simulink model "HmfCraneMbsModel"  (R2024b)
settings: Solver=FixedStepAuto  StartTime=0.0  StopTime=1  FixedStep=0.001  MaxStep=0.005  RelTol=1e-3
undefined symbols (not defined in the file): thetaList0, X, Y, Z
libraries: sm_lib x75, fl_lib x15, nesl_utility x12
(part 1 of 2)
settings Model: Creator=sindr  LastModifiedBy=hagen
settings RTWCC: GPUComputeCapability=3.5
settings ExplorerConfigSet: InternalSimMechanicsExplorerSettings="<ExplorerConfiguration><canonicalview>default</canonicalview><AnimationSetting><BasePlaybackSpeed>1.0</BasePlaybackSpeed><PlaybackSpeedFactor>1.0</PlaybackSpeedFactor></AnimationSetting><TilePanel><TileInfo><Tiles Columns=\"1\" Count=\"1\" Rows=\"1\"><Column Weight=\"1\"/><Row Weight=\"1\"/><Tile Height=\"1\" Width=\"1\" X=\"0\" Y=\"0\"/></Tiles></TileInfo><SceneInfo><SceneViewer><BGColor><R>0.800000011920928955</R><G>0.800000011920928955</G><B>0.800000011920928955</B></BGColor><Camera><DoPerspective>off</DoPerspective><Position><X>4.53532304319928414</X><Y>-3.6203597502527578</Y><Z>2.5915310173647752</Z></Position><Center><X>-0.318270324932377058</X><Y>2.33029046249896288</Y><Z>1.69505162107441443</Z></Center><Up><X>-0.0923543294804139991</X><Y>0.0742627373060478213</Y><Z>0.992953031957723553</Z></Up><ViewLimDist>1</ViewLimDist><YLim>4.99133206289738851</YLim><XLim>4.70316535078428188</XLim></Camera></SceneViewer></SceneInfo></TilePanel><MechEditorPanel><Cameras/><GfxPanelCameraMap/><VideoCreator><PlaybackSpeedRatio>1.0</PlaybackSpeedRatio><FrameRate>30</FrameRate><VideoFormat>Motion JPEG AVI</VideoFormat><FrameSize>auto</FrameSize></VideoCreator></MechEditorPanel></ExplorerConfiguration>"
settings ConfigComp: PLC_OutputDir=plc_export\FB_InverceKinematics  PLC_TargetIDE=twincat3  PLC_MultiTBSigbuilderTimeRange=off  PLC_FoldFBCallOutputVar=off  PLC_RemoveUnusedSSMethodCallArguments=off  PLC_UseCallOutputArgSyntax=off  PLC_EnableUnsignedAndDoubleTypes=off  PLC_EnableUDTSplitting=off  PLC_MaxFieldsInUDT=500  PLC_InlineEnumCastFunction=off

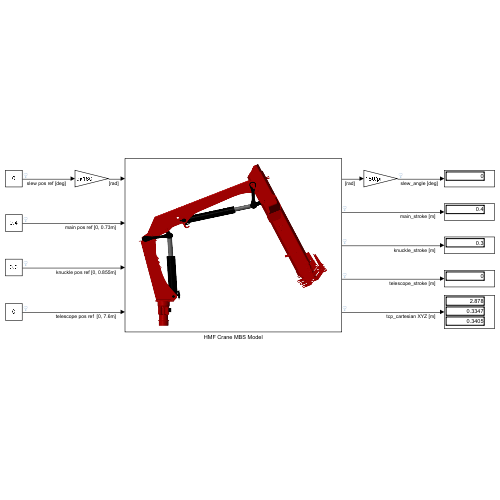
[thumbnail: Simulink's stored preview of the top-level diagram]
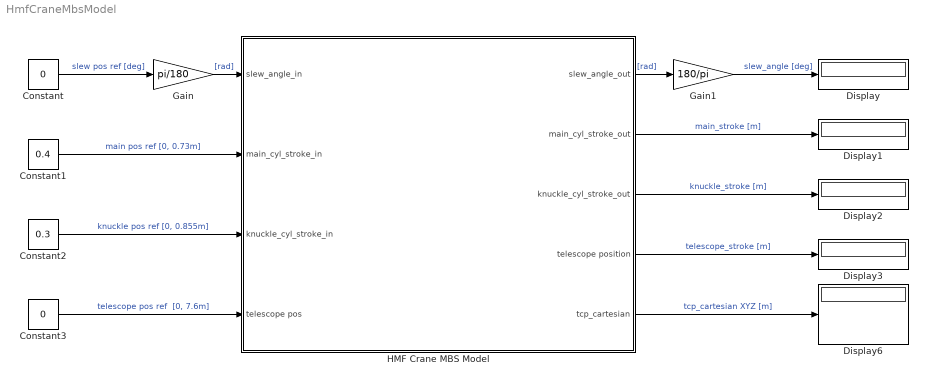
== system HmfCraneMbsModel ==
  Constant : Constant  Value=0
  Constant1 : Constant  Value=0.4
  Constant2 : Constant  Value=0.3
  Constant3 : Constant  Value=0
  Display{,1..3,6} (5 alike) : Display
  Gain : Gain  Gain=pi/180
  Gain1 : Gain  Gain=180/pi
  HMF Crane MBS Model : Subsystem
      mask Display: image('RedCraneMBS.png');
  wires:
  HMF Crane MBS Model/1(slew_angle_out) -> Gain1/1  "[rad]"
  HMF Crane MBS Model/2(main_cyl_stroke_out) -> Display1/1  "main_stroke [m]"
  HMF Crane MBS Model/3(knuckle_cyl_stroke_out) -> Display2/1  "knuckle_stroke [m]"
  HMF Crane MBS Model/4(telescope position) -> Display3/1  "telescope_stroke [m]"
  Constant/1 -> Gain/1  "slew pos ref [deg]"
  Constant1/1 -> HMF Crane MBS Model/2("main_cyl_stroke_in ")  "main pos ref [0, 0.73m]"
  Constant2/1 -> HMF Crane MBS Model/3(knuckle_cyl_stroke_in)  "knuckle pos ref [0, 0.855m]"
  Constant3/1 -> HMF Crane MBS Model/4(telescope pos)  "telescope pos ref  [0, 7.6m]"
  HMF Crane MBS Model/5(tcp_cartesian) -> Display6/1  "tcp_cartesian XYZ [m]"
  Gain/1 -> HMF Crane MBS Model/1(slew_angle_in)  "[rad]"
  Gain1/1 -> Display/1  "slew_angle [deg]"
